simulink model "EKF_OPT"  (R2024b)
settings: Solver=FixedStepAuto  StartTime=0.0  StopTime=250  FixedStep=0.05  RelTol=1e-3
values from neighbouring files (symbols this model uses):
  D = diag(dvec)    [singleRun.m]
undefined symbols (not defined in the file or in its folder): DiscIntNeverNeededParam, IRED, mRED, P_ic, x_ic, x_rel
libraries: slpidlib x6, simulink x2
(part 2 of 2)

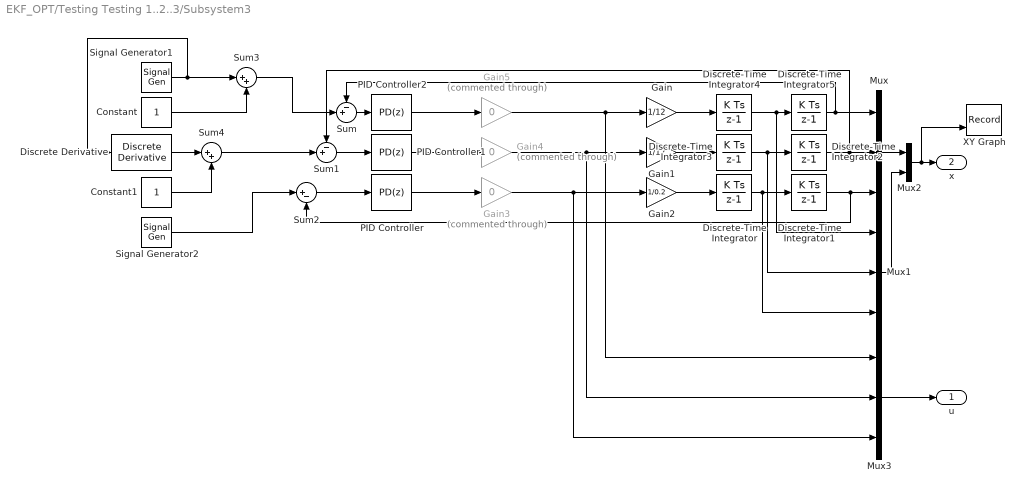
== system EKF_OPT/Testing Testing 1..2..3/Subsystem3 ==
  Constant : Constant
  Constant1 : Constant
  Discrete Derivative : simulink/Discrete/Discrete Derivative  gainval=1.0  ICPrevScaledInput=0.0  OutMin=[]  OutMax=[]  OutDataType=fixdt(1, 16)  OutScaling=2^-10  DoSatur=off
  Discrete-Time Integrator : DiscreteIntegrator  InitialCondition=-0.3  SampleTime=-1  ICPrevOutput=DiscIntNeverNeededParam  ICPrevScaledInput=DiscIntNeverNeededParam
  Discrete-Time Integrator1 : DiscreteIntegrator  SampleTime=-1  ICPrevOutput=DiscIntNeverNeededParam  ICPrevScaledInput=DiscIntNeverNeededParam
  Discrete-Time Integrator2 : DiscreteIntegrator  InitialCondition=2  SampleTime=-1  ICPrevOutput=DiscIntNeverNeededParam  ICPrevScaledInput=DiscIntNeverNeededParam
  Discrete-Time Integrator3 : DiscreteIntegrator  InitialCondition=0.2  SampleTime=-1  ICPrevOutput=DiscIntNeverNeededParam  ICPrevScaledInput=DiscIntNeverNeededParam
  Discrete-Time Integrator4 : DiscreteIntegrator  InitialCondition=-0.1  SampleTime=-1  ICPrevOutput=DiscIntNeverNeededParam  ICPrevScaledInput=DiscIntNeverNeededParam
  Discrete-Time Integrator5 : DiscreteIntegrator  InitialCondition=1  SampleTime=-1  ICPrevOutput=DiscIntNeverNeededParam  ICPrevScaledInput=DiscIntNeverNeededParam
  Gain : Gain  Gain=1/12
  Gain1 : Gain  Gain=1/12
  Gain2 : Gain  Gain=1/0.2
  Gain3 : Gain  Commented=through  Gain=0
  Gain4 : Gain  Commented=through  Gain=0
  Gain5 : Gain  Commented=through  Gain=0
  Mux : Mux  Inputs=3
  Mux1 : Mux  Inputs=3
  Mux2 : Mux  Inputs=2
  Mux3 : Mux  Inputs=3
  PID Controller : slpidlib/PID Controller  Controller=PD  Form=Parallel  TimeDomain=Discrete-time  UseExternalTs=off  SampleTime=-1  IntegratorMethod=Forward Euler  FilterMethod=Forward Euler  ControllerParametersSource=internal  P=0.00863228174020387  I=1  UseKiTs=off  D=0.441408383064275  UseExternalDerivativeSource=off  N=18.5475442531041  UseFilter=on  TunerSelectOption=Transfer Function Based (PID Tuner App)  InitialConditionSource=internal  InitialConditionForIntegrator=0  InitialConditionForFilter=0  DifferentiatorICPrevScaledInput=0  ExternalReset=none  TrackingMode=off  Kt=1  LimitOutput=off  SatLimitsSource=internal  UpperSaturationLimit=inf  LowerSaturationLimit=-inf  LinearizeAsGain=on  AntiWindupMode=none  Kb=1  LimitIntegrator=off  UpperIntegratorSaturationLimit=inf  LowerIntegratorSaturationLimit=-inf  POutMin=[]  POutMax=[]  IOutMin=[]  IOutMax=[]  DOutMin=[]  DOutMax=[]  NOutMin=[]  NOutMax=[]  SumOutMin=[]  SumOutMax=[]  SaturationOutMin=[]  SaturationOutMax=[]  PParamMin=[]  PParamMax=[]  IParamMin=[]  IParamMax=[]  DParamMin=[]  DParamMax=[]  NParamMin=[]  NParamMax=[]  KbParamMin=[]  KbParamMax=[]  KtParamMin=[]  KtParamMax=[]  KbOutMin=[]  KbOutMax=[]  KtOutMin=[]  KtOutMax=[]  IntegratorOutMin=[]  IntegratorOutMax=[]  FilterOutMin=[]  FilterOutMax=[]  SumI1OutMin=[]  SumI1OutMax=[]  SumI2OutMin=[]  SumI2OutMax=[]  SumI3OutMin=[]  SumI3OutMax=[]  SumI4OutMin=[]  SumI4OutMax=[]  SumDOutMin=[]  SumDOutMax=[]  DifferentiatorOutMin=[]  DifferentiatorOutMax=[]  FilterDiffOutCoefMin=[]  FilterDiffOutCoefMax=[]  ReciprocalOutMin=[]  ReciprocalOutMax=[]  SumDenOutMin=[]  SumDenOutMax=[]  SumNumOutMin=[]  SumNumOutMax=[]  DivideOutMin=[]  DivideOutMax=[]  UdiffTsProdOutMin=[]  UdiffTsProdOutMax=[]  NTsProdOutMin=[]  NTsProdOutMax=[]  UintegralTsProdOutMin=[]  UintegralTsProdOutMax=[]  UngainTsProdOutMin=[]  UngainTsProdOutMax=[]  ClampingZeroOutDataTypeStr=Inherit: Inherit via back propagation  ClampingZeroOutMin=[]  ClampingZeroOutMax=[]  FilterDenConstantOutDataTypeStr=Inherit: Inherit via back propagation  FilterDenConstantOutMin=[]  FilterDenConstantOutMax=[]  PCopyOutDataTypeStr=Inherit: Inherit via back propagation  PCopyOutMin=[]  PCopyOutMax=[]  NCopyOutDataTypeStr=Inherit: Inherit via back propagation  NCopyOutMin=[]  NCopyOutMax=[]  IntegratorContinuousStateAttributes=''  IntegratorStateMustResolveToSignalObject=off  IntegratorRTWStateStorageClass=Auto  FilterContinuousStateAttributes=''  FilterStateMustResolveToSignalObject=off  FilterRTWStateStorageClass=Auto  ParallelPVariant=InternalParameters  IdealPVariant=Disabled  IVariant=Disabled  DVariant=InternalParameters  IntegratorVariant=Disabled  SatVariant=Disabled  AWVariant=Disabled  PCopyVariant=Disabled  TRVariant=Disabled  FdbkBlocksVariant=Forward  IdealPFdbkVariant=Disabled  SatFdbkVariant=Disabled  DerivativeFilterVariant=ForwardEulerFilter  NVariant=InternalParameters  NCopyVariant=Disabled  FilterICVariant=InternalICsFilter  IntegratorICVariant=Disabled  ExternalResetVariant=Disabled  TRSumVariant=Passthrough  SumFdbkVariant=Disabled  SumVariant=Sum_PD  TsampFilterVariant=InternalTs  TsampNgainVariant=Passthrough  TsampIntegralVariant=Disabled_SignalSpec  ExternalSaturationOutDataTypeStr=Inherit: Same as second input  DerivativeSourceVariant=ErrorSignal  PreIntVariant=InternalPreInt
  PID Controller1 : slpidlib/PID Controller  Controller=PD  Form=Parallel  TimeDomain=Discrete-time  UseExternalTs=off  SampleTime=-1  IntegratorMethod=Forward Euler  FilterMethod=Forward Euler  ControllerParametersSource=internal  P=0.245018327394247  I=1  UseKiTs=off  D=18.2758094977982  UseExternalDerivativeSource=off  N=17.9496179817315  UseFilter=on  TunerSelectOption=Transfer Function Based (PID Tuner App)  InitialConditionSource=internal  InitialConditionForIntegrator=0  InitialConditionForFilter=0  DifferentiatorICPrevScaledInput=0  ExternalReset=none  TrackingMode=off  Kt=1  LimitOutput=off  SatLimitsSource=internal  UpperSaturationLimit=inf  LowerSaturationLimit=-inf  LinearizeAsGain=on  AntiWindupMode=none  Kb=1  LimitIntegrator=off  UpperIntegratorSaturationLimit=inf  LowerIntegratorSaturationLimit=-inf  POutMin=[]  POutMax=[]  IOutMin=[]  IOutMax=[]  DOutMin=[]  DOutMax=[]  NOutMin=[]  NOutMax=[]  SumOutMin=[]  SumOutMax=[]  SaturationOutMin=[]  SaturationOutMax=[]  PParamMin=[]  PParamMax=[]  IParamMin=[]  IParamMax=[]  DParamMin=[]  DParamMax=[]  NParamMin=[]  NParamMax=[]  KbParamMin=[]  KbParamMax=[]  KtParamMin=[]  KtParamMax=[]  KbOutMin=[]  KbOutMax=[]  KtOutMin=[]  KtOutMax=[]  IntegratorOutMin=[]  IntegratorOutMax=[]  FilterOutMin=[]  FilterOutMax=[]  SumI1OutMin=[]  SumI1OutMax=[]  SumI2OutMin=[]  SumI2OutMax=[]  SumI3OutMin=[]  SumI3OutMax=[]  SumI4OutMin=[]  SumI4OutMax=[]  SumDOutMin=[]  SumDOutMax=[]  DifferentiatorOutMin=[]  DifferentiatorOutMax=[]  FilterDiffOutCoefMin=[]  FilterDiffOutCoefMax=[]  ReciprocalOutMin=[]  ReciprocalOutMax=[]  SumDenOutMin=[]  SumDenOutMax=[]  SumNumOutMin=[]  SumNumOutMax=[]  DivideOutMin=[]  DivideOutMax=[]  UdiffTsProdOutMin=[]  UdiffTsProdOutMax=[]  NTsProdOutMin=[]  NTsProdOutMax=[]  UintegralTsProdOutMin=[]  UintegralTsProdOutMax=[]  UngainTsProdOutMin=[]  UngainTsProdOutMax=[]  ClampingZeroOutDataTypeStr=Inherit: Inherit via back propagation  ClampingZeroOutMin=[]  ClampingZeroOutMax=[]  FilterDenConstantOutDataTypeStr=Inherit: Inherit via back propagation  FilterDenConstantOutMin=[]  FilterDenConstantOutMax=[]  PCopyOutDataTypeStr=Inherit: Inherit via back propagation  PCopyOutMin=[]  PCopyOutMax=[]  NCopyOutDataTypeStr=Inherit: Inherit via back propagation  NCopyOutMin=[]  NCopyOutMax=[]  IntegratorContinuousStateAttributes=''  IntegratorStateMustResolveToSignalObject=off  IntegratorRTWStateStorageClass=Auto  FilterContinuousStateAttributes=''  FilterStateMustResolveToSignalObject=off  FilterRTWStateStorageClass=Auto  ParallelPVariant=InternalParameters  IdealPVariant=Disabled  IVariant=Disabled  DVariant=InternalParameters  IntegratorVariant=Disabled  SatVariant=Disabled  AWVariant=Disabled  PCopyVariant=Disabled  TRVariant=Disabled  FdbkBlocksVariant=Forward  IdealPFdbkVariant=Disabled  SatFdbkVariant=Disabled  DerivativeFilterVariant=ForwardEulerFilter  NVariant=InternalParameters  NCopyVariant=Disabled  FilterICVariant=InternalICsFilter  IntegratorICVariant=Disabled  ExternalResetVariant=Disabled  TRSumVariant=Passthrough  SumFdbkVariant=Disabled  SumVariant=Sum_PD  TsampFilterVariant=InternalTs  TsampNgainVariant=Passthrough  TsampIntegralVariant=Disabled_SignalSpec  ExternalSaturationOutDataTypeStr=Inherit: Same as second input  DerivativeSourceVariant=ErrorSignal  PreIntVariant=InternalPreInt
  PID Controller2 : slpidlib/PID Controller  Controller=PD  Form=Parallel  TimeDomain=Discrete-time  UseExternalTs=off  SampleTime=-1  IntegratorMethod=Forward Euler  FilterMethod=Forward Euler  ControllerParametersSource=internal  P=0.245018327394247  I=1  UseKiTs=off  D=18.2758094977982  UseExternalDerivativeSource=off  N=17.9496179817315  UseFilter=on  TunerSelectOption=Transfer Function Based (PID Tuner App)  InitialConditionSource=internal  InitialConditionForIntegrator=0  InitialConditionForFilter=0  DifferentiatorICPrevScaledInput=0  ExternalReset=none  TrackingMode=off  Kt=1  LimitOutput=off  SatLimitsSource=internal  UpperSaturationLimit=inf  LowerSaturationLimit=-inf  LinearizeAsGain=on  AntiWindupMode=none  Kb=1  LimitIntegrator=off  UpperIntegratorSaturationLimit=inf  LowerIntegratorSaturationLimit=-inf  POutMin=[]  POutMax=[]  IOutMin=[]  IOutMax=[]  DOutMin=[]  DOutMax=[]  NOutMin=[]  NOutMax=[]  SumOutMin=[]  SumOutMax=[]  SaturationOutMin=[]  SaturationOutMax=[]  PParamMin=[]  PParamMax=[]  IParamMin=[]  IParamMax=[]  DParamMin=[]  DParamMax=[]  NParamMin=[]  NParamMax=[]  KbParamMin=[]  KbParamMax=[]  KtParamMin=[]  KtParamMax=[]  KbOutMin=[]  KbOutMax=[]  KtOutMin=[]  KtOutMax=[]  IntegratorOutMin=[]  IntegratorOutMax=[]  FilterOutMin=[]  FilterOutMax=[]  SumI1OutMin=[]  SumI1OutMax=[]  SumI2OutMin=[]  SumI2OutMax=[]  SumI3OutMin=[]  SumI3OutMax=[]  SumI4OutMin=[]  SumI4OutMax=[]  SumDOutMin=[]  SumDOutMax=[]  DifferentiatorOutMin=[]  DifferentiatorOutMax=[]  FilterDiffOutCoefMin=[]  FilterDiffOutCoefMax=[]  ReciprocalOutMin=[]  ReciprocalOutMax=[]  SumDenOutMin=[]  SumDenOutMax=[]  SumNumOutMin=[]  SumNumOutMax=[]  DivideOutMin=[]  DivideOutMax=[]  UdiffTsProdOutMin=[]  UdiffTsProdOutMax=[]  NTsProdOutMin=[]  NTsProdOutMax=[]  UintegralTsProdOutMin=[]  UintegralTsProdOutMax=[]  UngainTsProdOutMin=[]  UngainTsProdOutMax=[]  ClampingZeroOutDataTypeStr=Inherit: Inherit via back propagation  ClampingZeroOutMin=[]  ClampingZeroOutMax=[]  FilterDenConstantOutDataTypeStr=Inherit: Inherit via back propagation  FilterDenConstantOutMin=[]  FilterDenConstantOutMax=[]  PCopyOutDataTypeStr=Inherit: Inherit via back propagation  PCopyOutMin=[]  PCopyOutMax=[]  NCopyOutDataTypeStr=Inherit: Inherit via back propagation  NCopyOutMin=[]  NCopyOutMax=[]  IntegratorContinuousStateAttributes=''  IntegratorStateMustResolveToSignalObject=off  IntegratorRTWStateStorageClass=Auto  FilterContinuousStateAttributes=''  FilterStateMustResolveToSignalObject=off  FilterRTWStateStorageClass=Auto  ParallelPVariant=InternalParameters  IdealPVariant=Disabled  IVariant=Disabled  DVariant=InternalParameters  IntegratorVariant=Disabled  SatVariant=Disabled  AWVariant=Disabled  PCopyVariant=Disabled  TRVariant=Disabled  FdbkBlocksVariant=Forward  IdealPFdbkVariant=Disabled  SatFdbkVariant=Disabled  DerivativeFilterVariant=ForwardEulerFilter  NVariant=InternalParameters  NCopyVariant=Disabled  FilterICVariant=InternalICsFilter  IntegratorICVariant=Disabled  ExternalResetVariant=Disabled  TRSumVariant=Passthrough  SumFdbkVariant=Disabled  SumVariant=Sum_PD  TsampFilterVariant=InternalTs  TsampNgainVariant=Passthrough  TsampIntegralVariant=Disabled_SignalSpec  ExternalSaturationOutDataTypeStr=Inherit: Same as second input  DerivativeSourceVariant=ErrorSignal  PreIntVariant=InternalPreInt
  Signal Generator1 : SignalGenerator  Frequency=2*pi/60  Units=rad/sec
  Signal Generator2 : SignalGenerator  Amplitude=0.01  Frequency=2*pi/60  Units=rad/sec
  Sum : Sum  Inputs=-+|
  Sum1 : Sum  Inputs=-+|
  Sum2 : Sum  Inputs=|+-
  Sum3 : Sum  Inputs=|++
  Sum4 : Sum  Inputs=|++
  XY Graph : Record  FileSettingsInternal="{\"entries\":[{\"content\":{\"excelSettings\":{\"content\":{},\"type\":\"Streamout.ExcelSettings\"}},\"type\":\"Streamout.FileSettingStorage\",\"uuid\":\"\"}],\"packageUris\":[\"http:\\/\\/schema.mathworks.com\\/mf0\\/streamout_blocks\\/R2020a\"],\"version\":\"1.0\"}"  Layout=[1 1]  SignalsInternal="{\"entries\":[{\"content\":{\"signals\":[{\"content\":{\"blockPath\":[],\"dimensions\":[1],\"domain\":\"\",\"lineColor\":\"#edb120\",\"lineWidth\":2,\"port\":1,\"signalID\":1},\"type\":\"RecordBlkView.Signal\",\"uuid\":\"\"},{\"content\":{\"blockPath\":[],\"dimensions\":[6],\"domain\":\"\",\"hasChildren\":true,\"lineColor\":\"#139fff\",\"lineWidth\":2,\"port\":2,\"signalID\":2,\"signalName\":\"Mux2\"},\"type\":\"RecordBlkView.Signal\",\"uuid\":\"\"},{\"content\":{\"blockPath\":[],\"channel\":[1],\"dimensions\":[6],\"domain\":\"\",\"lineColor\":\"#ff13a6\",\"lineWidth\":2,\"parentID\":2,\"port\":2,\"signalID\":3,\"signalName\":\"Mux2\"},\"type\":\"RecordBlkView.Signal\",\"uuid\":\"\"}]},\"type\":\"RecordBlkView.InputSignals\",\"uuid\":\"\"}],\"packageUris\":[\"http:\\/\\/schema.mathworks.com\\/mf0\\/streamout_blocks\\/R2020a\"],\"version\":\"1.0\"}"  VisualizationBindings="{\"xyplotplugin\":{\"info\":[{\"series\":[],\"subplotID\":1}]}}"  CompatibilityTag=XY
  u : Outport
  x : Outport  Port=2
  wires:
  Discrete-Time Integrator4/1 -> Discrete-Time Integrator5/1, Mux1/1
  Discrete-Time Integrator3/1 -> Discrete-Time Integrator2/1, Mux1/2
  Discrete-Time Integrator/1 -> Discrete-Time Integrator1/1, Mux1/3
  Discrete-Time Integrator1/1 -> Sum2/2, Mux/3
  Discrete-Time Integrator2/1 -> Mux/2, Sum1/1
  Discrete-Time Integrator5/1 -> Mux/1, Sum/1
  PID Controller2/1 -> Gain5/1
  PID Controller1/1 -> Gain4/1
  PID Controller/1 -> Gain3/1
  Mux/1 -> Mux2/1
  Mux1/1 -> Mux2/2
  Mux2/1 -> XY Graph/2, x/1
  Gain/1 -> Discrete-Time Integrator4/1
  Gain1/1 -> Discrete-Time Integrator3/1
  Gain2/1 -> Discrete-Time Integrator/1
  Mux3/1 -> u/1
  Sum/1 -> PID Controller2/1
  Sum2/1 -> PID Controller/1
  Sum1/1 -> PID Controller1/1
  Sum4/1 -> Sum1/2
  Constant/1 -> Sum3/2
  Signal Generator1/1 -> Discrete Derivative/1, Sum3/1
  Constant1/1 -> Sum4/2
  Discrete Derivative/1 -> Sum4/1
  Signal Generator2/1 -> Sum2/1
  Sum3/1 -> Sum/2
  Gain3/1 -> Mux3/3, Gain2/1
  Gain4/1 -> Gain1/1, Mux3/2
  Gain5/1 -> Gain/1, Mux3/1

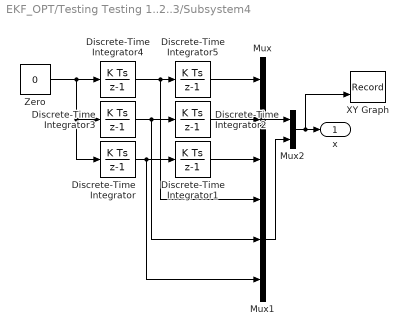
== system EKF_OPT/Testing Testing 1..2..3/Subsystem4 ==
  Discrete-Time Integrator : DiscreteIntegrator  InitialCondition=0.5  SampleTime=-1  ICPrevOutput=DiscIntNeverNeededParam  ICPrevScaledInput=DiscIntNeverNeededParam
  Discrete-Time Integrator1 : DiscreteIntegrator  InitialCondition=1  SampleTime=-1  ICPrevOutput=DiscIntNeverNeededParam  ICPrevScaledInput=DiscIntNeverNeededParam
  Discrete-Time Integrator2 : DiscreteIntegrator  InitialCondition=1  SampleTime=-1  ICPrevOutput=DiscIntNeverNeededParam  ICPrevScaledInput=DiscIntNeverNeededParam
  Discrete-Time Integrator3 : DiscreteIntegrator  InitialCondition=0.1  SampleTime=-1  ICPrevOutput=DiscIntNeverNeededParam  ICPrevScaledInput=DiscIntNeverNeededParam
  Discrete-Time Integrator4 : DiscreteIntegrator  InitialCondition=0.1  SampleTime=-1  ICPrevOutput=DiscIntNeverNeededParam  ICPrevScaledInput=DiscIntNeverNeededParam
  Discrete-Time Integrator5 : DiscreteIntegrator  InitialCondition=1  SampleTime=-1  ICPrevOutput=DiscIntNeverNeededParam  ICPrevScaledInput=DiscIntNeverNeededParam
  Mux : Mux  Inputs=3
  Mux1 : Mux  Inputs=3
  Mux2 : Mux  Inputs=2
  XY Graph : Record  FileSettingsInternal="{\"entries\":[{\"content\":{\"excelSettings\":{\"content\":{},\"type\":\"Streamout.ExcelSettings\"}},\"type\":\"Streamout.FileSettingStorage\",\"uuid\":\"\"}],\"packageUris\":[\"http:\\/\\/schema.mathworks.com\\/mf0\\/streamout_blocks\\/R2020a\"],\"version\":\"1.0\"}"  Layout=[1 1]  SignalsInternal="{\"entries\":[{\"content\":{\"signals\":[{\"content\":{\"blockPath\":[],\"dimensions\":[1],\"domain\":\"\",\"lineColor\":\"#7e2f8e\",\"lineWidth\":2,\"port\":1,\"signalID\":1},\"type\":\"RecordBlkView.Signal\",\"uuid\":\"\"},{\"content\":{\"blockPath\":[],\"dimensions\":[6],\"domain\":\"\",\"hasChildren\":true,\"lineColor\":\"#b746ff\",\"lineWidth\":2,\"port\":2,\"signalID\":2,\"signalName\":\"Mux2\"},\"type\":\"RecordBlkView.Signal\",\"uuid\":\"\"},{\"content\":{\"blockPath\":[],\"channel\":[1],\"dimensions\":[6],\"domain\":\"\",\"lineColor\":\"#22b573\",\"lineWidth\":2,\"parentID\":2,\"port\":2,\"signalID\":3,\"signalName\":\"Mux2\"},\"type\":\"RecordBlkView.Signal\",\"uuid\":\"\"}]},\"type\":\"RecordBlkView.InputSignals\",\"uuid\":\"\"}],\"packageUris\":[\"http:\\/\\/schema.mathworks.com\\/mf0\\/streamout_blocks\\/R2020a\"],\"version\":\"1.0\"}"  VisualizationBindings="{\"xyplotplugin\":{\"info\":[{\"series\":[],\"subplotID\":1}]}}"  CompatibilityTag=XY
  Zero : Constant  Value=0  OutDataTypeStr=Inherit: Inherit via back propagation
  x : Outport
  wires:
  Discrete-Time Integrator4/1 -> Discrete-Time Integrator5/1, Mux1/1
  Discrete-Time Integrator3/1 -> Discrete-Time Integrator2/1, Mux1/2
  Discrete-Time Integrator/1 -> Discrete-Time Integrator1/1, Mux1/3
  Discrete-Time Integrator1/1 -> Mux/3
  Discrete-Time Integrator2/1 -> Mux/2
  Discrete-Time Integrator5/1 -> Mux/1
  Mux/1 -> Mux2/1
  Mux1/1 -> Mux2/2
  Mux2/1 -> XY Graph/2, x/1
  Zero/1 -> Discrete-Time Integrator/1, Discrete-Time Integrator3/1, Discrete-Time Integrator4/1

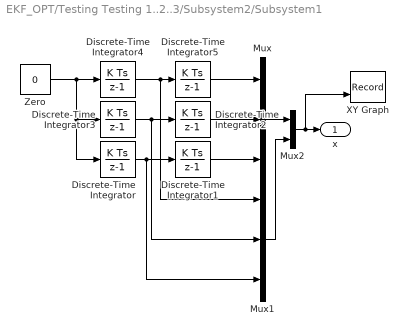
== system EKF_OPT/Testing Testing 1..2..3/Subsystem2/Subsystem1 ==
  Discrete-Time Integrator : DiscreteIntegrator  InitialCondition=0.5  SampleTime=-1  ICPrevOutput=DiscIntNeverNeededParam  ICPrevScaledInput=DiscIntNeverNeededParam
  Discrete-Time Integrator1 : DiscreteIntegrator  InitialCondition=1  SampleTime=-1  ICPrevOutput=DiscIntNeverNeededParam  ICPrevScaledInput=DiscIntNeverNeededParam
  Discrete-Time Integrator2 : DiscreteIntegrator  InitialCondition=1  SampleTime=-1  ICPrevOutput=DiscIntNeverNeededParam  ICPrevScaledInput=DiscIntNeverNeededParam
  Discrete-Time Integrator3 : DiscreteIntegrator  InitialCondition=0.1  SampleTime=-1  ICPrevOutput=DiscIntNeverNeededParam  ICPrevScaledInput=DiscIntNeverNeededParam
  Discrete-Time Integrator4 : DiscreteIntegrator  InitialCondition=0.1  SampleTime=-1  ICPrevOutput=DiscIntNeverNeededParam  ICPrevScaledInput=DiscIntNeverNeededParam
  Discrete-Time Integrator5 : DiscreteIntegrator  InitialCondition=1  SampleTime=-1  ICPrevOutput=DiscIntNeverNeededParam  ICPrevScaledInput=DiscIntNeverNeededParam
  Mux : Mux  Inputs=3
  Mux1 : Mux  Inputs=3
  Mux2 : Mux  Inputs=2
  XY Graph : Record  FileSettingsInternal="{\"entries\":[{\"content\":{\"excelSettings\":{\"content\":{},\"type\":\"Streamout.ExcelSettings\"}},\"type\":\"Streamout.FileSettingStorage\",\"uuid\":\"\"}],\"packageUris\":[\"http:\\/\\/schema.mathworks.com\\/mf0\\/streamout_blocks\\/R2020a\"],\"version\":\"1.0\"}"  Layout=[1 1]  SignalsInternal="{\"entries\":[{\"content\":{},\"type\":\"RecordBlkView.InputSignals\",\"uuid\":\"\"}],\"packageUris\":[\"http:\\/\\/schema.mathworks.com\\/mf0\\/streamout_blocks\\/R2020a\"],\"version\":\"1.0\"}"  VisualizationBindings="{\"xyplotplugin\":{\"info\":[{\"series\":[],\"subplotID\":1}]}}"  CompatibilityTag=XY
  Zero : Constant  Value=0  OutDataTypeStr=Inherit: Inherit via back propagation
  x : Outport
  wires:
  Discrete-Time Integrator4/1 -> Discrete-Time Integrator5/1, Mux1/1
  Discrete-Time Integrator3/1 -> Discrete-Time Integrator2/1, Mux1/2
  Discrete-Time Integrator/1 -> Discrete-Time Integrator1/1, Mux1/3
  Discrete-Time Integrator1/1 -> Mux/3
  Discrete-Time Integrator2/1 -> Mux/2
  Discrete-Time Integrator5/1 -> Mux/1
  Mux/1 -> Mux2/1
  Mux1/1 -> Mux2/2
  Mux2/1 -> XY Graph/2, x/1
  Zero/1 -> Discrete-Time Integrator/1, Discrete-Time Integrator3/1, Discrete-Time Integrator4/1

== system EKF_OPT/Testing Testing 1..2..3/Subsystem2/noise ==
  Mux : Mux  Inputs=3
  Random Number : RandomNumber  Variance=0.05^2  Seed=789235  SampleTime=0.1
  Random Number1 : RandomNumber  Variance=0.05^2  Seed=34257  SampleTime=0.1
  Random Number2 : RandomNumber  Variance=0.05^2  Seed=431260  SampleTime=0.1
  Out1 : Outport
  wires:
  Random Number/1 -> Mux/1
  Random Number1/1 -> Mux/2
  Random Number2/1 -> Mux/3
  Mux/1 -> Out1/1

== system EKF_OPT/Testing Testing 1..2..3/Subsystem2/noise1 ==
  Mux : Mux  Inputs=3
  Random Number : RandomNumber  Variance=0.05^2  Seed=1239746  SampleTime=0.1
  Random Number1 : RandomNumber  Variance=0.05^2  Seed=182347  SampleTime=0.1
  Random Number2 : RandomNumber  Variance=0.05^2  Seed=123456  SampleTime=0.1
  Out1 : Outport
  wires:
  Mux/1 -> Out1/1
  Random Number2/1 -> Mux/3
  Random Number1/1 -> Mux/2
  Random Number/1 -> Mux/1

== system EKF_OPT/Testing Testing 1..2..3/Subsystem2/noise2 ==
  Mux : Mux  Inputs=3
  Random Number : RandomNumber  Variance=0.1^2  Seed=672589  SampleTime=0.1
  Random Number1 : RandomNumber  Variance=0.1^2  Seed=12304967  SampleTime=0.1
  Random Number2 : RandomNumber  Variance=0.1^2  Seed=234908  SampleTime=0.1
  Out1 : Outport
  wires:
  Random Number/1 -> Mux/1
  Random Number1/1 -> Mux/2
  Random Number2/1 -> Mux/3
  Mux/1 -> Out1/1

== matlab function EKF_OPT/Testing Testing 1..2..3/MATLAB Function2 ==
  data: proc input; x_PS output
function x_PS = fcn(proc)

x_PS = proc(1:6);
end

== matlab function EKF_OPT/Testing Testing 1..2..3/MATLAB Function3 ==
  data: x_old input; angles input; u input; x_new output
function x_new = Euler(x_old, angles, u)
m = 12;
J = 0.2;
dt = 0.001;

theta_s = angles(1);
w_s = angles(2);

dx = relativeDynamics(x_old, theta_s, w_s, u, m, J);

x_new = x_old + dt*dx;

end


function dx = relativeDynamics(x_rel, theta_s, w_s, u, m_s, J_s)
% relativeDynamics  Compute 3-DOF relative rates in servicer frame
%
% Inputs:
%   x_rel : 6x1 relative state [x; y; theta; vx; vy; omega]
%   theta_s : servicer attitude (rad)
%   w_s   : servicer angular rate (rad/s)
%   u     : 3x1 control input [u1; u2; u3]
%           u1,u2 = inertial-frame forces (Fx, Fy)
%           u3 = inertial-frame torque (about z)
%   m_s   : servicer mass
%   J_s   : servicer moment of inertia
%
% Output:
%   dx    : 6x1 derivative of [x; y; theta; vx; vy; omega]

% Extract states
r_rel     = x_rel(1:2);    % relative position [x; y]
v_rel     = x_rel(4:5);    % relative velocity [vx; vy]
omega_rel = x_rel(6);      % relative angular rate

% Rotation from inertial to servicer body frame
R_s = [ cos(theta_s),  sin(theta_s);
       -sin(theta_s),  cos(theta_s) ];

% Skew-symmetric for z-axis
S = [0, -1; 1, 0];

% —— Kinematics: position derivative in rotating frame —— 
% v_rel = v_rel + w_s * (S * r_rel);

% Compute servicer accelerations in its body frame
a_s_body = R_s * (u(1:2)/m_s);  % linear accel in body frame
alpha_s  = u(3)/J_s;            % angular accel (scalar)

% Relative linear acceleration (transport theorem)
a_rel = - a_s_body ...             % servicer thrust
      - 2*w_s*(S * v_rel) ...      % Coriolis
      - alpha_s*(S * r_rel) ...    % angular accel effect
      + w_s^2 * r_rel;             % centripetal

% Relative angular acceleration
alpha_rel = - alpha_s;

% Pack derivatives
dx = [ v_rel;                  % x_dot, y_dot
       omega_rel;              % theta_dot
       a_rel;                  % vx_dot, vy_dot
       alpha_rel ];            % omega_dot
end

== matlab function EKF_OPT/Testing Testing 1..2..3/MATLAB Function1 ==
  data: proc input; CNN output; LiDAR output; LRF output
function [CNN, LiDAR, LRF] = fcn(proc)

CNN = proc(7:10);
LiDAR = proc(11:14);
LRF = proc(15);

== matlab function EKF_OPT/Testing Testing 1..2..3/MATLAB Function5 ==
  data: rel_vec input; LOS_vec output
function LOS_vec = rel2LOS(rel_vec)
    x = rel_vec(1);
    y = rel_vec(2);

    p = sqrt(x^2 + y^2);

    u = rel_vec(1:2)/p;

    LOS_vec = [u; p; rel_vec(3)];

end

== matlab function EKF_OPT/Testing Testing 1..2..3/MATLAB Function4 ==
  data: u input; y output
function y = fcn(u)

y = u([3,6]);

== matlab function EKF_OPT/Subsystem2/NaN_Hold/MATLAB Function ==
  data: u_curr input; y output; u_prev input
function y = fcn(u_curr, u_prev)

if sum(abs(u_curr-u_prev)) > 10^-10
    y = nan(size(u_curr));
else
    y = u_curr;
end

== matlab function EKF_OPT/Subsystem2/NaN_Hold1/MATLAB Function ==
  data: u_curr input; y output; u_prev input
function y = fcn(u_curr, u_prev)

if sum(abs(u_curr-u_prev)) > 10^-10
    y = nan(size(u_curr));
else
    y = u_curr;
end

== matlab function EKF_OPT/Subsystem2/NaN_Hold2/MATLAB Function ==
  data: u_curr input; y output; u_prev input
function y = fcn(u_curr, u_prev)

if sum(abs(u_curr-u_prev)) > 10^-10
    y = nan(size(u_curr));
else
    y = u_curr;
end

== matlab function EKF_OPT/Testing Testing 1..2..3/MATLAB Function6 ==
  data: x_s input; x_rel output; x_c input
function x_rel = globalToRelative(x_s, x_c)
% globalToRelative  Compute relative state in servicer frame
%
% Inputs:
%   x_s : 6x1 servicer global state [x_s; y_s; theta_s; dx_s; dy_s; dtheta_s]
%   x_c : 6x1 client  global state [x_c; y_c; theta_c; dx_c; dy_c; dtheta_c]
%
% Output:
%   x_rel : 6x1 relative state [x_rel; y_rel; theta_rel; vx_rel; vy_rel; omega_rel]

% Extract positions and orientations
r_s      = x_s(1:2);
r_c      = x_c(1:2);
theta_s  = x_s(3);
theta_c  = x_c(3);

% Extract velocities
dr_s     = x_s(4:5);
dr_c     = x_c(4:5);
w_s      = x_s(6);
w_c      = x_c(6);

% Rotation matrix from inertial to servicer frame
R_s = [cos(theta_s),  sin(theta_s);
       -sin(theta_s), cos(theta_s)];

% Skew-symmetric matrix in 2D
S = [0, -1; 1, 0];

% Relative position in servicer frame
r_rel = R_s*(r_c - r_s);

% Relative orientation
theta_rel = theta_c - theta_s;

% Relative velocity in servicer frame (transport theorem)
v_rel = R_s*(dr_c - dr_s) - w_s*(S*r_rel);

% Relative angular rate
omega_rel = w_c - w_s;

% Assemble relative state
x_rel = [
    r_rel;           % [x_rel; y_rel]
    theta_rel;       % theta_rel
    v_rel;           % [vx_rel; vy_rel]
    omega_rel       % omega_rel
];
end

== matlab function EKF_OPT/Testing Testing 1..2..1/MATLAB Function ==
  data: ref_traj output; t input
function ref_traj = fcn(t)
% x_rel : 6x1 relative state [x; y; theta; vx; vy; omega]
x = 0.75; % in track circle
y = 0; % Along Track
dx = 0;
dy = 0;
w_t = 2*pi/60;
theta = w_t*t;

ref_traj = [x; y; theta; dx; dy; w_t];

== matlab function EKF_OPT/Testing Testing 1..2..1/LQR+FeedForward/Feed Forward ==
  data: x_rel input; u input; F_sum output
function F_sum  = Euler(x_rel, u)
% relativeDynamics  Compute 3-DOF relative rates in servicer frame
%
% Inputs:
%   x_rel : 8x1 relative state [x; y; theta; vx; vy; omega, theta_frame, omega_frame]
%   u     : 3x1 control input Body frame [u1; u2; u3]
%           u1,u2 = Body-frame forces (Fx, Fy)
%           u3 = Body-frame torque (about z)
%   m_s   : servicer mass
%   J_s   : servicer moment of inertia
%
% Output:
%   F     : Feedforward force

m = 12;
J = 0.2;

% Extract states
r_rel     = x_rel(1:2);    % relative position [x; y]
v_rel     = x_rel(4:5);    % relative velocity [vx; vy]
omega_rel = x_rel(6);      % relative angular rate
theta_s   = x_rel(7);      % Frame Angle
w_s       = x_rel(8);      % Frame rotation rate

F_sum = u;

% Skew-symmetric for z-axis
S = [0, -1; 1, 0];

% Compute servicer accelerations in its body frame
alpha_s  = u(3)/J;            % angular accel (scalar)

a_cor  = - 2*w_s*(S * v_rel);     % Coriolis
a_cent = - alpha_s*(S * r_rel);   % angular accel effect
a_acc  = w_s^2 * r_rel;           % centripetal

% Apply negative acceleration to remove non-inertial terms
F_sum(1:2) = F_sum(1:2) - m*(a_cor + a_cent + a_acc);

end

== matlab function EKF_OPT/Testing Testing 1..2..1/MATLAB Function3 ==
  data: x_old input; u input; x_new output
function x_new = Euler(x_old, u)
m = 12;
J = 0.2;
dt = 0.001;

% % Rotation from inertial to servicer body frame
% R_s = [ cos(theta_s),  sin(theta_s);
%        -sin(theta_s),  cos(theta_s) ];
% 
% u_body = u;
% u_body(1:2) = R_s*u(1:2);

dx = relativeDynamics(x_old, u, m, J);

x_new = x_old + dt*dx;

end


function dx = relativeDynamics(x_rel, u, m_s, J_s)
% relativeDynamics  Compute 3-DOF relative rates in servicer frame
%
% Inputs:
%   x_rel : 8x1 relative state [x; y; theta; vx; vy; omega, theta_frame, omega_frame]
%   u     : 3x1 control input Body frame [u1; u2; u3]
%           u1,u2 = Body-frame forces (Fx, Fy)
%           u3 = Body-frame torque (about z)
%   m_s   : servicer mass
%   J_s   : servicer moment of inertia
%
% Output:
%   dx    : 6x1 derivative of [x; y; theta; vx; vy; omega, theta_frame, omega_frame]

% Extract states
r_rel     = x_rel(1:2);    % relative position [x; y]
v_rel     = x_rel(4:5);    % relative velocity [vx; vy]
omega_rel = x_rel(6);      % relative angular rate
theta_s   = x_rel(7);      % Frame Angle
w_s       = x_rel(8);      % Frame rotation rate

% Skew-symmetric for z-axis
S = [0, -1; 1, 0];

% Compute servicer accelerations in its body frame
a_s_body = (u(1:2)/m_s);  % linear accel in body frame
alpha_s  = u(3)/J_s;            % angular accel (scalar)

% Relative linear acceleration (transport theorem)
a_rel = a_s_body ...             % servicer thrust
      - 2*w_s*(S * v_rel) ...      % Coriolis
      - alpha_s*(S * r_rel) ...    % angular accel effect
      + w_s^2 * r_rel;             % centripetal

% Relative angular acceleration
alpha_rel = - alpha_s;

% Pack derivatives
dx = [ v_rel;                  % x_dot, y_dot
       omega_rel;              % theta_dot
       a_rel;                  % vx_dot, vy_dot
       alpha_rel;              % omega_dot
       w_s;
       alpha_s];  

end

== matlab function EKF_OPT/Testing Testing 1..2..1/LQR+FeedForward/LQR ==
  data: err input; F output
function F = fcn(err)
% m = 12;
% J = 0.2;
% M = [1/m,1/m,1/J];
% 
% A = [zeros(3), eye(3);
%      zeros(3), zeros(3)];
% 
% B = [zeros(3);
%      diag(M)];
% 
% sys = ss(A,B,[],[]);
% 
% dt = 1;
% G = [(0.5*dt^2)*eye(3);
%      dt*eye(3)];
% 
% q = 10;
% r = 1;
% 
% Q = G*q*G';
% R = r*diag(M);
% 
% K = lqr(sys,Q,R);

% K = [5.47722557505166	-4.93585577850187e-15	-1.86244783899409e-15	15.8572826739401	3.33066907387547e-15	-3.26744418108217e-15;
% 1.13173575156928e-15	5.47722557505167	6.32373002387479e-16	1.04816158538957e-15	15.8572826739401	-8.46269022761931e-16;
% 3.10248778947243e-16	-7.32141592448225e-17	0.707106781186548	6.39311302790644e-16	-1.61396183681627e-16	1.51090790999141];

K = [diag([0.1, 0.1, 0.001]), diag([1, 1, 0.01])];
F = K*err;

== matlab function EKF_OPT/Testing Testing 1..2..1/LQR+FeedForward/MATLAB Function ==
  data: u input; y output
function y = fcn(u)
% remove uncontrollable states

y = [u(1); ... x
     u(2); ... y
     u(7); ... theta
     u(4); ... dx
     u(5); ... dy
     u(8);]; % dthteta

== matlab function EKF_OPT/Testing Testing 1..2..3/MATLAB Function7 ==
  data: x_old input; u input; x_new output
function x_new = Euler(x_old, u)
m = 12;
J = 0.2;
dt = 0.001;

% % Rotation from inertial to servicer body frame
% R_s = [ cos(theta_s),  sin(theta_s);
%        -sin(theta_s),  cos(theta_s) ];
% 
% u_body = u;
% u_body(1:2) = R_s*u(1:2);

dx = relativeDynamics(x_old, u, m, J);

x_new = x_old + dt*dx;

end


function dx = relativeDynamics(x_rel, u, m_s, J_s)
% relativeDynamics  Compute 3-DOF relative rates in servicer frame
%
% Inputs:
%   x_rel : 6x1 relative state [x; y; theta; vx; vy; omega]
%   u     : 3x1 control input Body frame [u1; u2; u3]
%           u1,u2 = inertial-frame forces (Fx, Fy)
%           u3 = inertial-frame torque (about z)
%   m_s   : servicer mass
%   J_s   : servicer moment of inertia
%
% Output:
%   dx    : 6x1 derivative of [x; y; theta; vx; vy; omega]

% Extract states
r_rel     = x_rel(1:2);    % relative position [x; y]
v_rel     = x_rel(4:5);    % relative velocity [vx; vy]
omega_rel = x_rel(6);      % relative angular rate
theta_s   = x_rel(7);      % Frame Angle
w_s       = x_rel(8);      % Frame rotation rate

% Skew-symmetric for z-axis
S = [0, -1; 1, 0];

% —— Kinematics: position derivative in rotating frame —— 
% v_rel = v_rel + w_s * (S * r_rel);

% Compute servicer accelerations in its body frame
a_s_body = (u(1:2)/m_s);        % linear accel in body frame
alpha_s  = u(3)/J_s;            % angular accel (scalar)

% Relative linear acceleration (transport theorem)
a_rel = - a_s_body ...             % servicer thrust
      - 2*w_s*(S * v_rel) ...      % Coriolis
      - alpha_s*(S * r_rel) ...    % angular accel effect
      + w_s^2 * r_rel;             % centripetal

% Relative angular acceleration
alpha_rel = - alpha_s;

% Pack derivatives
dx = [ v_rel;                  % x_dot, y_dot
       omega_rel;              % theta_dot
       a_rel;                  % vx_dot, vy_dot
       alpha_rel;              % omega_dot
       w_s;
       alpha_s];            
end

== matlab function EKF_OPT/Testing Testing 1..2..3/MATLAB Function8 ==
  data: theta input; u input; u_body output
function u_body = fcn(theta, u)

theta_s = theta(3);

% Rotation from inertial to servicer body frame
R_s = [ cos(theta_s),  sin(theta_s);
       -sin(theta_s),  cos(theta_s) ];

u_body = u;
u_body(1:2) = R_s*u(1:2);

== matlab function EKF_OPT/Testing Testing 1..2..1/LQR+FeedForward/MATLAB Function1 ==
  data: true input; ref input; u output
function u = fcn(true, ref)

== matlab function EKF_OPT/MATLAB Function ==
  data: xStack input; x_INS output; x_GNS output; x_fuse output; PEst input
function [x_INS, x_GNS, x_fuse] = fcn(xStack, PEst)

[x_INS, ~, x_GNS, ~, x_fuse, ~] = TempFilterModule.Misc.unpackStates(xStack, PEst);

== matlab function EKF_OPT/Subsystem2/NaN_Hold3/MATLAB Function ==
  data: u_curr input; y output; u_prev input
function y = fcn(u_curr, u_prev)

if sum(abs(u_curr-u_prev)) > 10^-10
    y = nan(size(u_curr));
else
    y = u_curr;
end

== matlab function EKF_OPT/SpotEstimator1 ==
  data: phase input; proc input; cmd input; est output; est_vel output; paramEst parameter; est_bias output; debug output
function [est,est_vel,est_bias,debug] = SpotEstimator(phase, proc, cmd, paramEst)

    [est,est_vel,est_bias,debug] = SpotEstimator(phase, proc, cmd, paramEst);

end

== matlab function EKF_OPT/Subsystem/MATLAB Function3 ==
  data: xStack input; x_INS output; P_INS output; x_GNS output; P_GNS output; x_fuse output; PEst input; P_fuse output
function [x_INS, P_INS, x_GNS, P_GNS, x_fuse, P_fuse] = fcn(xStack, PEst)

[x_INS, P_INS, x_GNS, P_GNS, x_fuse, P_fuse] = TempFilterModule.Misc.unpackStates(xStack, PEst);

== matlab function EKF_OPT/Subsystem1/MATLAB Function ==
  data: proc input; x_PS output; LOS_Stereo output; LOS_LiDAR output; LRF output; IMU output
function [x_PS, LOS_Stereo, LOS_LiDAR, LRF, IMU] = fcn(proc)
%% Data Processing
red = proc([SpotSensor.xRedPhasespace; ...
            SpotSensor.yRedPhasespace; ...
            SpotSensor.thetaRedPhasespace; ...
            SpotSensor.xRedRatePhasespace; ...
            SpotSensor.yRedRatePhasespace; ...
            SpotSensor.thetaRedRatePhasespace]);

black = proc([SpotSensor.xBlackPhasespace; ...
              SpotSensor.yBlackPhasespace; ...
              SpotSensor.thetaBlackPhasespace; ...
              SpotSensor.xBlackRatePhasespace; ...
              SpotSensor.yBlackRatePhasespace; ...
              SpotSensor.thetaBlackRatePhasespace]);

theta_s = red(3);

x_PS = [globalToRelative(red, black); red(3,1); red(6,1)];

Stereo = proc([SpotSensor.xStereo; ...
            SpotSensor.yStereo; ...
            SpotSensor.thetaStereo]);

LOS_Stereo = rel2LOS(Stereo);

LiDAR = proc([SpotSensor.xLidar; ...
              SpotSensor.yLidar; ...
              SpotSensor.thetaLidar]);
LOS_LiDAR = rel2LOS(LiDAR);

LRF = proc(SpotSensor.rLaser);

IMU = [theta_s; proc(SpotSensor.thetaRedImu)];

end

function x_rel = globalToRelative(x_s, x_c)
% globalToRelative  Compute relative state in servicer frame
%
% Inputs:
%   x_s : 6x1 servicer global state [x_s; y_s; theta_s; dx_s; dy_s; dtheta_s]
%   x_c : 6x1 client  global state [x_c; y_c; theta_c; dx_c; dy_c; dtheta_c]
%
% Output:
%   x_rel : 6x1 relative state [x_rel; y_rel; theta_rel; vx_rel; vy_rel; omega_rel]

% Extract positions and orientations
r_s      = x_s(1:2);
r_c      = x_c(1:2);
theta_s  = x_s(3);
theta_c  = x_c(3);

% Extract velocities
dr_s     = x_s(4:5);
dr_c     = x_c(4:5);
w_s      = x_s(6);
w_c      = x_c(6);

% Rotation matrix from inertial to servicer frame
R_s = [cos(theta_s),  sin(theta_s);
       -sin(theta_s), cos(theta_s)];

% Skew-symmetric matrix in 2D
S = [0, -1; 1, 0];

% Relative position in servicer frame
r_rel = R_s*(r_c - r_s);

% Relative orientation
theta_rel = theta_c - theta_s;

% Relative velocity in servicer frame (transport theorem)
v_rel = R_s*(dr_c - dr_s) - w_s*(S*r_rel);

% Relative angular rate
omega_rel = w_c - w_s;

% Assemble relative state
x_rel = [
    r_rel;           % [x_rel; y_rel]
    theta_rel;       % theta_rel
    v_rel;           % [vx_rel; vy_rel]
    omega_rel       % omega_rel
];
end

function LOS_vec = rel2LOS(rel_vec)
    x = rel_vec(1);
    y = rel_vec(2);

    p = sqrt(x^2 + y^2);

    u = rel_vec(1:2)/p;

    LOS_vec = [u; p; rel_vec(3)];

end

== matlab function EKF_OPT/MATLAB Function1 ==
  data: t input; phase output; paramPhaseMgmt parameter
function phase  = SpotPhaseMgmt(t, paramPhaseMgmt)

    [phase] = SpotPhaseMgmt(t, paramPhaseMgmt);

end

== matlab function EKF_OPT/Subsystem/MATLAB Function ==
  data: u input; proc input; t input; xStack input; PStack input; xStack output; PStack output; navOpts parameter; bias output; d output; V output
function [xStack, PStack, bias, d, V] = fcn( u, proc, t, xStack, PStack, navOpts)
%% Data Processing
red = proc([SpotSensor.xRedPhasespace; ...
            SpotSensor.yRedPhasespace; ...
            SpotSensor.thetaRedPhasespace; ...
            SpotSensor.xRedRatePhasespace; ...
            SpotSensor.yRedRatePhasespace; ...
            SpotSensor.thetaRedRatePhasespace]);

black = proc([SpotSensor.xBlackPhasespace; ...
              SpotSensor.yBlackPhasespace; ...
              SpotSensor.thetaBlackPhasespace; ...
              SpotSensor.xBlackRatePhasespace; ...
              SpotSensor.yBlackRatePhasespace; ...
              SpotSensor.thetaBlackRatePhasespace]);

% if t >= 35.56
%     disp('here')
% end

theta_s = red(3);

% Rotation from inertial to servicer body frame
R_s = [ cos(theta_s),  sin(theta_s);
       -sin(theta_s),  cos(theta_s) ];

u(1:2) = R_s'*u(1:2);

xrelPS = globalToRelative(red, black);

Stereo = proc([SpotSensor.xStereo; ...
            SpotSensor.yStereo; ...
            SpotSensor.thetaStereo]);

LOS_Stereo = rel2LOS(Stereo);

LiDAR = proc([SpotSensor.xLidar; ...
              SpotSensor.yLidar; ...
              SpotSensor.thetaLidar]);
LOS_LiDAR = rel2LOS(LiDAR);

LRF = proc(SpotSensor.rLaser);

IMU = [theta_s; proc(SpotSensor.thetaRedImu)];

x_PS = [xrelPS(1:3); IMU];
% x_PS = [xrelPS(1:3); red([3,6],1)];
% x_PS = nan(size(x_PS));
LOS_Stereo = nan(size(LOS_Stereo));
% LOS_LiDAR = nan(size(LOS_LiDAR));
LRF = nan(size(LRF));
% IMU = nan(size(IMU));

sensors = [LOS_Stereo; LOS_LiDAR; LRF; IMU];

dt = 0.05;

% if navOpts.OLR
%     disp(u)
% end
%% Call Filter Module 
[xStack, PStack, EKFout] = TempFilterModule.EstimateStates(xStack, PStack, u, dt, x_PS, sensors, navOpts);
% xStack = xStack;
% PStack = PStack;

bias = [EKFout.SageHusa.r_LRF; % 1
        EKFout.SageHusa.r_IMU; % 2,3
        EKFout.SageHusa.r_Lidar; % 4, 5, 6, 7
        EKFout.SageHusa.r_Stereo; % 8, 9, 10, 11
        EKFout.SageHusa.r_PS;]; % 12, 13, 14, 15, 16
d = EKFout.EKF_INS.d;

V = EKFout.EKF_INS.V;
% bias = -EKFout.SageHusa.r_IMU;
% bias = [0;0];
end

function LOS_vec = rel2LOS(rel_vec)
    x = rel_vec(1);
    y = rel_vec(2);

    p = sqrt(x^2 + y^2);

    u = rel_vec(1:2)/p;

    LOS_vec = [u; p; rel_vec(3)];

end

function x_rel = globalToRelative(x_s, x_c)
% globalToRelative  Compute relative state in servicer frame
%
% Inputs:
%   x_s : 6x1 servicer global state [x_s; y_s; theta_s; dx_s; dy_s; dtheta_s]
%   x_c : 6x1 client  global state [x_c; y_c; theta_c; dx_c; dy_c; dtheta_c]
%
% Output:
%   x_rel : 6x1 relative state [x_rel; y_rel; theta_rel; vx_rel; vy_rel; omega_rel]

% Extract positions and orientations
r_s      = x_s(1:2);
r_c      = x_c(1:2);
theta_s  = x_s(3);
theta_c  = x_c(3);

% Extract velocities
dr_s     = x_s(4:5);
dr_c     = x_c(4:5);
w_s      = x_s(6);
w_c      = x_c(6);

% Rotation matrix from inertial to servicer frame
R_s = [cos(theta_s),  sin(theta_s);
       -sin(theta_s), cos(theta_s)];

% Skew-symmetric matrix in 2D
S = [0, -1; 1, 0];

% Relative position in servicer frame
r_rel = R_s*(r_c - r_s);

% Relative orientation
theta_rel = theta_c - theta_s;

% Relative velocity in servicer frame (transport theorem)
v_rel = R_s*(dr_c - dr_s) - w_s*(S*r_rel);

% Relative angular rate
omega_rel = w_c - w_s;

% Assemble relative state
x_rel = [
    r_rel;           % [x_rel; y_rel]
    theta_rel;       % theta_rel
    v_rel;           % [vx_rel; vy_rel]
    omega_rel       % omega_rel
];
end

== matlab function EKF_OPT/Force/MATLAB Function1 ==
  data: u input; y output; mRED parameter; IRED parameter
function y = fcn(u, mRED, IRED)

y = u;

y(1:2) = y(1:2)*mRED;

y(3) = y(3)*IRED;

== matlab function EKF_OPT/MATLAB Function4 ==
  data: proc input; LOS_CNN output; LOS_LiDAR output; LRF output
function [LOS_CNN, LOS_LiDAR, LRF] = fcn(proc)

CNN = proc([SpotSensor.xStereo; ...
            SpotSensor.yStereo; ...
            SpotSensor.thetaStereo]);

LOS_CNN = rel2LOS(CNN);

LiDAR = proc([SpotSensor.xLidar; ...
              SpotSensor.yLidar; ...
              SpotSensor.thetaLidar]);

LOS_LiDAR = rel2LOS(LiDAR);

LRF = proc(SpotSensor.rLaser);

end

function LOS_vec = rel2LOS(rel_vec)
    x = rel_vec(1);
    y = rel_vec(2);

    p = sqrt(x^2 + y^2);

    u = rel_vec(1:2)/p;

    LOS_vec = [u; p; rel_vec(3)];

end

== matlab function EKF_OPT/MATLAB Function5 ==
  data: rel_vec_3D input; LOS_vec output
function LOS_vec = rel2LOS(rel_vec_3D)
    rel_vec = rel_vec_3D(:,1,1);
    x = rel_vec(1);
    y = rel_vec(2);

    p = sqrt(x^2 + y^2);

    u = rel_vec(1:2)/p;

    LOS_vec = [u; p; rel_vec(3)];

end

== matlab function EKF_OPT/Testing Testing 1..2..3/MATLAB Function ==
  data: x_prev input; P_prev input; red input; u input; x_est output; sensors input; P_est output; sensormode output
function [x_est, P_est, sensormode] = fcn(x_prev, P_prev, red, u, sensors)
%% Data Processing

% sensors = [x_PS; LOS_CNN; LOS_LiDAR; LRF];
sensors = nan(size(sensors));
%% Initialize - Not Tuned
params.w_s = red(6);
params.theta_s = red(3);
params.m_s = 12;
params.J_s = 0.2;

navOpts.Q = 0.001*eye(3);
navOpts.R_PS = 0.000001*eye(3);
navOpts.R_Rn = 0.1;
navOpts.R_CNN = 0.001*eye(4);
navOpts.R_LiDAR = 0.01*eye(4);
navOpts.OLR = false;
navOpts.dmax = 3;
navOpts.params = params;

dt = 0.01;

%% Call Filter Module 

[x_est, P_est, sensormode] = TempFilterModule.EstimateStates(x_prev, P_prev, u, dt, sensors, navOpts);
% x_est = x_prev;
% P_est = P_prev;
% sensormode = 1;
end

function LOS_vec = rel2LOS(rel_vec)
    x = rel_vec(1);
    y = rel_vec(2);

    p = sqrt(x^2 + y^2);

    u = rel_vec(1:2)/p;

    LOS_vec = [u; p; rel_vec(3)];

end

function x_rel = globalToRelative(x_s, x_c)
% globalToRelative  Compute relative state in servicer frame
%
% Inputs:
%   x_s : 6x1 servicer global state [x_s; y_s; theta_s; dx_s; dy_s; dtheta_s]
%   x_c : 6x1 client  global state [x_c; y_c; theta_c; dx_c; dy_c; dtheta_c]
%
% Output:
%   x_rel : 6x1 relative state [x_rel; y_rel; theta_rel; vx_rel; vy_rel; omega_rel]

% Extract positions and orientations
r_s      = x_s(1:2);
r_c      = x_c(1:2);
theta_s  = x_s(3);
theta_c  = x_c(3);

% Extract velocities
dr_s     = x_s(4:5);
dr_c     = x_c(4:5);
w_s      = x_s(6);
w_c      = x_c(6);

% Rotation matrix from inertial to servicer frame
R_s = [cos(theta_s),  sin(theta_s);
       -sin(theta_s), cos(theta_s)];

% Skew-symmetric matrix in 2D
S = [0, -1; 1, 0];

% Relative position in servicer frame
r_rel = R_s*(r_c - r_s);

% Relative orientation
theta_rel = theta_c - theta_s;

% Relative velocity in servicer frame (transport theorem)
v_rel = R_s*(dr_c - dr_s) - w_s*(S*r_rel);

% Relative angular rate
omega_rel = w_c - w_s;

% Assemble relative state
x_rel = [
    r_rel;           % [x_rel; y_rel]
    theta_rel;       % theta_rel
    v_rel;           % [vx_rel; vy_rel]
    omega_rel       % omega_rel
];
end

== matlab function EKF_OPT/Testing Testing 1..2..3/Subsystem2/Sensor Models ==
  data: black input; red input; sensors output; noiseCNN input; noiseLiDAR input; noiseLRF input; CNN output; LiDAR output
function [sensors, CNN, LiDAR] = fcn(black, red, noiseCNN, noiseLiDAR, noiseLRF)

x_PS = globalToRelative(red, black);

CNN = x_PS(1:3) + noiseCNN;
LOS_CNN = rel2LOS(CNN);

LiDAR = x_PS(1:3) + noiseLiDAR;
LOS_LiDAR = rel2LOS(LiDAR);

LRF_temp = x_PS(1:3) + noiseLRF;
LOS_LRF_temp = rel2LOS(LRF_temp);
LRF = LOS_LRF_temp(4);

sensors = [x_PS; LOS_CNN; LOS_LiDAR; LRF];

end

function LOS_vec = rel2LOS(rel_vec)
    x = rel_vec(1);
    y = rel_vec(2);

    p = sqrt(x^2 + y^2);

    u = rel_vec(1:2)/p;

    LOS_vec = [u; p; rel_vec(3)];

end

function x_rel = globalToRelative(x_s, x_c)
% globalToRelative  Compute relative state in servicer frame
%
% Inputs:
%   x_s : 6x1 servicer global state [x_s; y_s; theta_s; dx_s; dy_s; dtheta_s]
%   x_c : 6x1 client  global state [x_c; y_c; theta_c; dx_c; dy_c; dtheta_c]
%
% Output:
%   x_rel : 6x1 relative state [x_rel; y_rel; theta_rel; vx_rel; vy_rel; omega_rel]

% Extract positions and orientations
r_s      = x_s(1:2);
r_c      = x_c(1:2);
theta_s  = x_s(3);
theta_c  = x_c(3);

% Extract velocities
dr_s     = x_s(4:5);
dr_c     = x_c(4:5);
w_s      = x_s(6);
w_c      = x_c(6);

% Rotation matrix from inertial to servicer frame
R_s = [cos(theta_s),  sin(theta_s);
       -sin(theta_s), cos(theta_s)];

% Skew-symmetric matrix in 2D
S = [0, -1; 1, 0];

% Relative position in servicer frame
r_rel = R_s*(r_c - r_s);

% Relative orientation
theta_rel = theta_c - theta_s;

% Relative velocity in servicer frame (transport theorem)
v_rel = R_s*(dr_c - dr_s) - w_s*(S*r_rel);

% Relative angular rate
omega_rel = w_c - w_s;

% Assemble relative state
x_rel = [
    r_rel;           % [x_rel; y_rel]
    theta_rel;       % theta_rel
    v_rel;           % [vx_rel; vy_rel]
    omega_rel       % omega_rel
];
end
